simulink model "Luanvancu"  (R2018a)
settings: Solver=ode4  StartTime=0.0  StopTime=500  FixedStep=0.1  RelTol=1e-3
libraries: simulink x2
settings Model: EnablePacing=on  Creator=Hungs  LastModifiedBy=Hungs
settings DataIOCC: SaveOutput=off  SignalLogging=off  DSMLogging=off  SaveTime=off

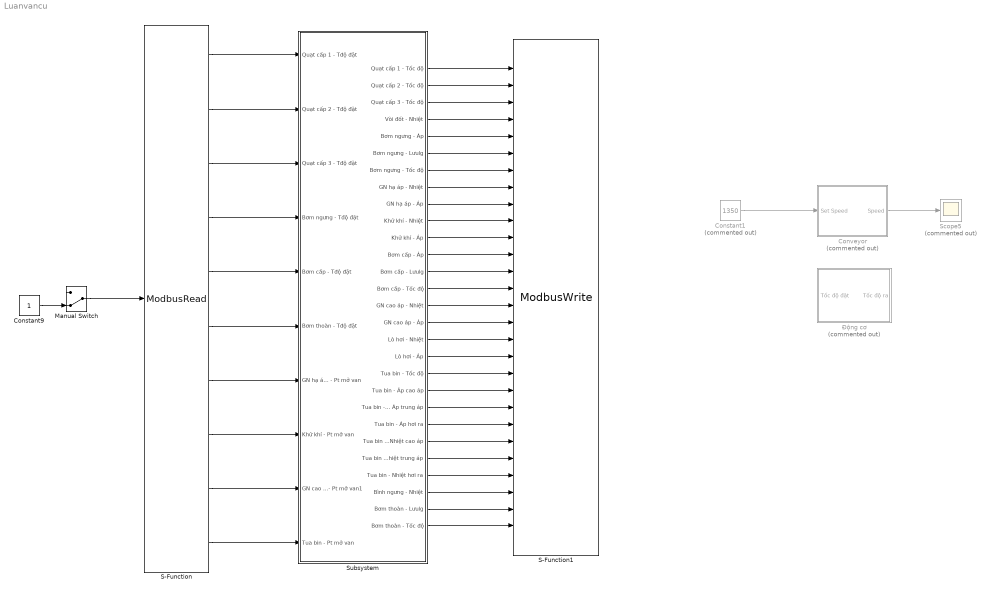
== system Luanvancu ==
  Constant1 : Constant  Commented=on  Value=1350
  Constant9 : Constant
  Conveyor : Subsystem  Commented=on
      mask Display: image('C:\Program Files\MATLAB\ThermalElectricity\Maskicon\conveyor.png');
  Manual Switch : ManualSwitch  CurrentSetting=0
  S-Function : S-Function  FunctionName=ModbusRead  Parameters='127.0.0.1' 502  SFunctionDeploymentMode=off  EnableBusSupport=off
  S-Function1 : S-Function  FunctionName=ModbusWrite  Parameters='127.0.0.1' 502  SFunctionDeploymentMode=off  EnableBusSupport=off
  Scope5 : Scope  Commented=on
  Subsystem : Subsystem
  Động cơ : Subsystem  Commented=on
  wires:
  Constant1/1 -> Conveyor/1(Set Speed)
  Conveyor/1(Speed) -> Scope5/1
  Manual Switch/1 -> S-Function/1
  Constant9/1 -> Manual Switch/2
  S-Function/1 -> Subsystem/1(Quạt cấp 1 - Tđộ đặt)
  S-Function/2 -> Subsystem/2(Quạt cấp 2 - Tđộ đặt)
  S-Function/3 -> Subsystem/3(Quạt cấp 3 - Tđộ đặt)
  S-Function/4 -> Subsystem/4(Bơm ngưng - Tđộ đặt)
  S-Function/5 -> Subsystem/5(Bơm cấp - Tđộ đặt)
  S-Function/6 -> Subsystem/6(Bơm thoàn - Tđộ đặt)
  S-Function/7 -> Subsystem/7(GN hạ áp - Pt mở van)
  S-Function/8 -> Subsystem/8(Khử khí - Pt mở van)
  S-Function/9 -> Subsystem/9(GN cao áp - Pt mở van1)
  S-Function/10 -> Subsystem/10(Tua bin - Pt mở van)
  Subsystem/1(Quạt cấp 1 - Tốc độ) -> S-Function1/1
  Subsystem/2(Quạt cấp 2 - Tốc độ) -> S-Function1/2
  Subsystem/3(Quạt cấp 3 - Tốc độ) -> S-Function1/3
  Subsystem/4(Vòi đốt - Nhiệt) -> S-Function1/4
  Subsystem/5(Bơm ngưng - Áp) -> S-Function1/5
  Subsystem/6(Bơm ngưng - Lưulg) -> S-Function1/6
  Subsystem/7(Bơm ngưng - Tốc độ) -> S-Function1/7
  Subsystem/8(GN hạ áp - Nhiệt) -> S-Function1/8
  Subsystem/9(GN hạ áp - Áp) -> S-Function1/9
  Subsystem/10(Khử khí - Nhiệt) -> S-Function1/10
  Subsystem/11(Khử khí - Áp) -> S-Function1/11
  Subsystem/12(Bơm cấp - Áp) -> S-Function1/12
  Subsystem/13(Bơm cấp - Lưulg) -> S-Function1/13
  Subsystem/14(Bơm cấp - Tốc độ) -> S-Function1/14
  Subsystem/15(GN cao áp - Nhiệt) -> S-Function1/15
  Subsystem/16(GN cao áp - Áp) -> S-Function1/16
  Subsystem/17(Lò hơi - Nhiệt) -> S-Function1/17
  Subsystem/18(Lò hơi - Áp) -> S-Function1/18
  Subsystem/19(Tua bin - Tốc độ) -> S-Function1/19
  Subsystem/20(Tua bin - Áp cao áp) -> S-Function1/20
  Subsystem/21(Tua bin - Áp trung áp) -> S-Function1/21
  Subsystem/22(Tua bin - Áp hơi ra) -> S-Function1/22
  Subsystem/23(Tua bin - Nhiệt cao áp) -> S-Function1/23
  Subsystem/24(Tua bin - Nhiệt trung áp) -> S-Function1/24
  Subsystem/25(Tua bin - Nhiệt hơi ra) -> S-Function1/25
  Subsystem/26(Bình ngưng - Nhiệt) -> S-Function1/26
  Subsystem/27(Bơm thoàn - Lưulg) -> S-Function1/27
  Subsystem/28(Bơm thoàn - Tốc độ) -> S-Function1/28

== system Luanvancu/Conveyor ==
  Set Speed : Inport
  Motor_1 : TransferFcn  Denominator=[1 1 1]
  Speed : Outport
  wires:
  Set Speed/1 -> Motor_1/1
  Motor_1/1 -> Speed/1

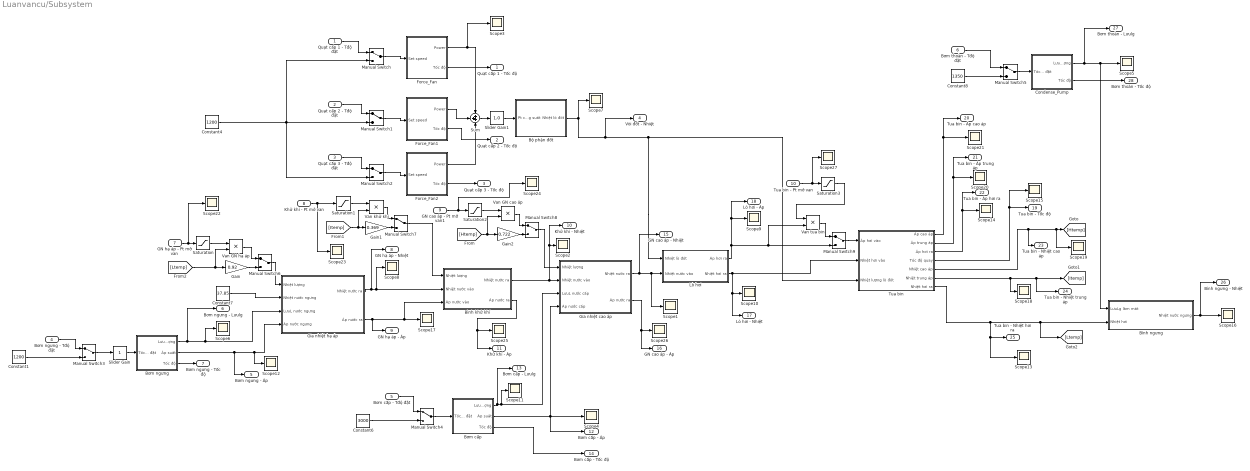
== system Luanvancu/Subsystem ==
  Quạt cấp 1 - Tđộ đặt : Inport
  Quạt cấp 2 - Tđộ đặt : Inport  Port=2
  Quạt cấp 3 - Tđộ đặt : Inport  Port=3
  Bơm ngưng - Tđộ đặt : Inport  Port=4
  Bơm cấp - Tđộ đặt : Inport  Port=5
  Bơm thoàn - Tđộ đặt : Inport  Port=6
  GN hạ áp - Pt mở van : Inport  Port=7
  Khử khí - Pt mở van : Inport  Port=8
  GN cao áp - Pt mở van1 : Inport  Port=9
  Tua bin - Pt mở van : Inport  Port=10
  Bình khử khí : Subsystem
  Bình ngưng : Subsystem
  Bơm cấp : Subsystem
      mask Display: image('C:\Program Files\MATLAB\ThermalElectricity\Maskicon\Pump.png');
  Bơm ngưng : Subsystem
      mask Display: image('C:\Program Files\MATLAB\ThermalElectricity\Maskicon\Pump.png');
  Bộ phận đốt : Subsystem
      mask Display: image('C:\Program Files\MATLAB\ThermalElectricity\Maskicon\Furnace.png');
  Condense_Pump : Subsystem
      mask Display: image('C:\Program Files\MATLAB\ThermalElectricity\Maskicon\Pump.png');
  Constant1 : Constant  Value=1200
  Constant4 : Constant  Value=1200
  Constant6 : Constant  Value=3000
  Constant7 : Constant  Value=37.85
  Constant8 : Constant  Value=1350
  Force_Fan : Subsystem
      mask Display: image('C:\Program Files\MATLAB\ThermalElectricity\Maskicon\Fan.png');
  Force_Fan1 : Subsystem
      mask Display: image('C:\Program Files\MATLAB\ThermalElectricity\Maskicon\Fan.png');
  Force_Fan2 : Subsystem
      mask Display: image('C:\Program Files\MATLAB\ThermalElectricity\Maskicon\Fan.png');
  Gain : Gain  Gain=0.92
  Gain1 : Gain  Gain=0.369
  Gain2 : Gain  Gain=0.722
  Gia nhiệt cao áp : Subsystem
  Gia nhiệt hạ áp : Subsystem
  Lò hơi : Subsystem
  Manual Switch{,1..9} (10 alike) : ManualSwitch
  Saturation{,1..3} (4 alike) : Saturate  UpperLimit=1  LowerLimit=0
  Scope{1..27} (27 alike) : Scope
  Slider Gain : simulink/Math Operations/Slider Gain  gain=1  low=0  high=2
  Slider Gain1 : simulink/Math Operations/Slider Gain  gain=1.0  low=0  high=2
  Sum : Sum  Inputs=+++
  Tua bin : Subsystem
  Van GN cao áp : Product
  Van GN hạ áp : Product
  Van khử khí : Product
  Van tua bin : Product
  Quạt cấp 1 - Tốc độ : Outport
  Quạt cấp 2 - Tốc độ : Outport  Port=2
  Quạt cấp 3 - Tốc độ : Outport  Port=3
  Vòi đốt - Nhiệt : Outport  Port=4
  Bơm ngưng - Áp : Outport  Port=5
  Bơm ngưng - Lưulg : Outport  Port=6
  Bơm ngưng - Tốc độ : Outport  Port=7
  GN hạ áp - Nhiệt : Outport  Port=8
  GN hạ áp - Áp : Outport  Port=9
  Khử khí - Nhiệt : Outport  Port=10
  Khử khí - Áp : Outport  Port=11
  Bơm cấp - Áp : Outport  Port=12
  Bơm cấp - Lưulg : Outport  Port=13
  Bơm cấp - Tốc độ : Outport  Port=14
  GN cao áp - Nhiệt : Outport  Port=15
  GN cao áp - Áp : Outport  Port=16
  Lò hơi - Nhiệt : Outport  Port=17
  Lò hơi - Áp : Outport  Port=18
  Tua bin - Tốc độ : Outport  Port=19
  Tua bin - Áp cao áp : Outport  Port=20
  Tua bin - Áp trung áp : Outport  Port=21
  Tua bin - Áp hơi ra : Outport  Port=22
  Tua bin - Nhiệt cao áp : Outport  Port=23
  Tua bin - Nhiệt trung áp : Outport  Port=24
  Tua bin - Nhiệt hơi ra : Outport  Port=25
  Bình ngưng - Nhiệt : Outport  Port=26
  Bơm thoàn - Lưulg : Outport  Port=27
  Bơm thoàn - Tốc độ : Outport  Port=28
  wires:
  Gia nhiệt cao áp/2(Áp nước ra) -> GN cao áp - Áp/1, Scope26/1
  Slider Gain1/1 -> Bộ phận đốt/1(Pt công suất)
  Sum/1 -> Slider Gain1/1
  Constant7/1 -> Gia nhiệt hạ áp/2(Nhiệt nước ngưng)
  Force_Fan/1(Power) -> Sum/1, Scope3/1
  Force_Fan1/1(Power) -> Sum/2
  Gia nhiệt hạ áp/2(Áp nước ra) -> GN hạ áp - Áp/1, Scope17/1, Bình khử khí/3(Áp nước vào)
  Lò hơi/1(Áp hơi ra) -> Lò hơi - Áp/1, Scope9/1, Manual Switch9/2, Van tua bin/2
  Bộ phận đốt/1(Nhiệt lò đốt) -> Vòi đốt - Nhiệt/1, Lò hơi/1(Nhiệt lò đốt), Tua bin/3(Nhiệt lượng lò đốt), Scope7/1
  Tua bin/3(Áp hơi ra) -> Tua bin - Áp hơi ra/1, Scope14/1
  Bình ngưng/1(Nhiệt nước ngưng) -> Bình ngưng - Nhiệt/1, Scope16/1
  Slider Gain/1 -> Bơm ngưng/1(Tốc độ đặt)
  Condense_Pump/1(Lưu lượng) -> Bơm thoàn - Lưulg/1, Bình ngưng/1(LưuLg làm mát), Scope5/1
  Bình khử khí/2(Áp nước ra) -> Khử khí - Áp/1, Scope25/1
  Tua bin/4(Tốc độ quay) -> Scope15/1, Tua bin - Tốc độ/1
  Manual Switch/1 -> Force_Fan/1(Set speed)
  Quạt cấp 1 - Tđộ đặt/1 -> Manual Switch/1
  Quạt cấp 2 - Tđộ đặt/1 -> Manual Switch1/1
  Manual Switch2/1 -> Force_Fan2/1(Set speed)
  Manual Switch1/1 -> Force_Fan1/1(Set speed)
  Quạt cấp 3 - Tđộ đặt/1 -> Manual Switch2/1
  Manual Switch3/1 -> Slider Gain/1
  Bơm ngưng - Tđộ đặt/1 -> Manual Switch3/1
  Manual Switch4/1 -> Bơm cấp/1(Tốc độ đặt)
  Bơm cấp - Tđộ đặt/1 -> Manual Switch4/1
  Manual Switch5/1 -> Condense_Pump/1(Tốc độ đặt)
  Constant8/1 -> Manual Switch5/2
  Bơm thoàn - Tđộ đặt/1 -> Manual Switch5/1
  Tua bin/6(Nhiệt trung áp) -> Scope18/1, Tua bin - Nhiệt trung áp/1, [Itemp]
  Tua bin/5(Nhiệt cao áp) -> Tua bin - Nhiệt cao áp/1, Scope19/1, [Htemp]
  [Ltemp] -> Van GN hạ áp/2, Gain/1
  Saturation/1 -> Van GN hạ áp/1
  Saturation1/1 -> Van khử khí/1
  [Htemp] -> Van GN cao áp/2, Gain2/1
  Saturation3/1 -> Van tua bin/1
  [Itemp] -> Van khử khí/2, Gain1/1
  Tua bin/7(Nhiệt hơi ra) -> Bình ngưng/2(Nhiệt hơi), [Ltemp], Scope13/1, Tua bin - Nhiệt hơi ra/1
  Bơm ngưng/1(Lưu lượng) -> Gia nhiệt hạ áp/3(LưuL nước ngưng), Scope6/1, Bơm ngưng - Lưulg/1
  Manual Switch6/1 -> Gia nhiệt hạ áp/1(Nhiệt lượng)
  Van GN hạ áp/1 -> Manual Switch6/1
  Manual Switch7/1 -> Bình khử khí/1(Nhiệt lượng)
  Van khử khí/1 -> Manual Switch7/1
  Manual Switch8/1 -> Gia nhiệt cao áp/1(Nhiệt lượng)
  Van GN cao áp/1 -> Manual Switch8/1
  Manual Switch9/1 -> Tua bin/1(Áp hơi vào)
  Van tua bin/1 -> Manual Switch9/1
  Bơm cấp/1(Lưu lượng) -> Bơm cấp - Lưulg/1, Scope11/1, Gia nhiệt cao áp/3(LưuL nước cấp)
  Gain/1 -> Manual Switch6/2
  Gain1/1 -> Manual Switch7/2
  Gain2/1 -> Manual Switch8/2
  Lò hơi/2(Nhiệt hơi ra) -> Lò hơi - Nhiệt/1, Scope10/1, Tua bin/2(Nhiệt hơi vào)
  Bơm ngưng/3(Tốc độ) -> Bơm ngưng - Tốc độ/1
  Bơm cấp/3(Tốc độ) -> Bơm cấp - Tốc độ/1
  Condense_Pump/2(Tốc độ) -> Bơm thoàn - Tốc độ/1
  Tua bin/2(Áp trung áp) -> Tua bin - Áp trung áp/1, Scope20/1
  Tua bin/1(Áp cao áp) -> Tua bin - Áp cao áp/1, Scope21/1
  Force_Fan2/1(Power) -> Sum/3
  Force_Fan2/2(Tốc độ) -> Quạt cấp 3 - Tốc độ/1
  Force_Fan1/2(Tốc độ) -> Quạt cấp 2 - Tốc độ/1
  Force_Fan/2(Tốc độ) -> Quạt cấp 1 - Tốc độ/1
  GN hạ áp - Pt mở van/1 -> Scope22/1, Saturation/1
  Bơm ngưng/2(Áp suất) -> Bơm ngưng - Áp/1, Scope12/1, Gia nhiệt hạ áp/4(Áp nước ngưng)
  Constant1/1 -> Manual Switch3/2
  Bơm cấp/2(Áp suất) -> Bơm cấp - Áp/1, Gia nhiệt cao áp/4(Áp nước cấp), Scope4/1
  Constant6/1 -> Manual Switch4/2
  Bình khử khí/1(Nhiệt nước ra) -> Khử khí - Nhiệt/1, Scope2/1, Gia nhiệt cao áp/2(Nhiệt nước vào)
  Gia nhiệt hạ áp/1(Nhiệt nước ra) -> GN hạ áp - Nhiệt/1, Bình khử khí/2(Nhiệt nước vào), Scope8/1
  Constant4/1 -> Manual Switch2/2, Manual Switch1/2, Manual Switch/2
  Gia nhiệt cao áp/1(Nhiệt nước ra) -> GN cao áp - Nhiệt/1, Scope1/1, Lò hơi/2(Nhiệt nước vào)
  Saturation2/1 -> Van GN cao áp/1
  GN cao áp - Pt mở van1/1 -> Scope24/1, Saturation2/1
  Khử khí - Pt mở van/1 -> Scope23/1, Saturation1/1
  Tua bin - Pt mở van/1 -> Scope27/1, Saturation3/1

== system Luanvancu/Động cơ ==
  Tốc độ đặt : Inport
  Bão hòa 2 cực : Saturate  UpperLimit=1500  LowerLimit=0
  Động cơ AC : TransferFcn  Denominator=[1 1 1]
  Tốc độ ra : Outport
  wires:
  Bão hòa 2 cực/1 -> Tốc độ ra/1
  Tốc độ đặt/1 -> Động cơ AC/1
  Động cơ AC/1 -> Bão hòa 2 cực/1

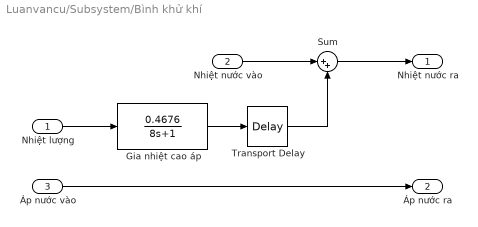
== system Luanvancu/Subsystem/Bình khử khí ==
  Nhiệt lượng : Inport
  Nhiệt nước vào : Inport  Port=2
  Áp nước vào : Inport  Port=3
  Gia nhiệt cao áp : TransferFcn  Numerator=[0.4676]  Denominator=[8 1]
  Sum : Sum  Inputs=|++
  Transport Delay : TransportDelay  DelayTime=3
  Nhiệt nước ra : Outport
  Áp nước ra : Outport  Port=2
  wires:
  Nhiệt lượng/1 -> Gia nhiệt cao áp/1
  Nhiệt nước vào/1 -> Sum/1
  Gia nhiệt cao áp/1 -> Transport Delay/1
  Sum/1 -> Nhiệt nước ra/1
  Áp nước vào/1 -> Áp nước ra/1
  Transport Delay/1 -> Sum/2

== system Luanvancu/Subsystem/Bình ngưng ==
  LưuLg làm mát : Inport
  Nhiệt hơi : Inport  Port=2
  Constant8 : Constant  Value=37.85
  Ngưng tụ : TransferFcn  Numerator=[6.883]  Denominator=[12 1]
  Sum : Sum  Inputs=|+-
  Sum1 : Sum  Inputs=|++
  Transport Delay : TransportDelay  DelayTime=3
  Nhiệt nước ngưng : Outport
  wires:
  Ngưng tụ/1 -> Transport Delay/1
  Nhiệt hơi/1 -> Sum/1
  LưuLg làm mát/1 -> Ngưng tụ/1
  Sum/1 -> Sum1/1
  Sum1/1 -> Nhiệt nước ngưng/1
  Constant8/1 -> Sum1/2
  Transport Delay/1 -> Sum/2

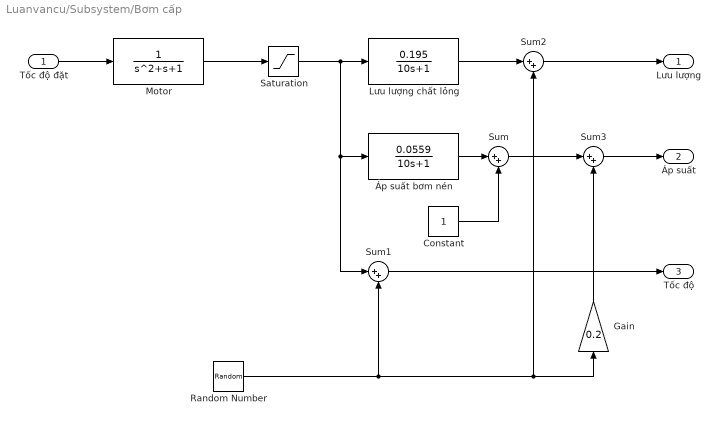
== system Luanvancu/Subsystem/Bơm cấp ==
  Tốc độ đặt : Inport
  Constant : Constant
  Gain : Gain  Gain=0.2
  Lưu lượng chất lỏng : TransferFcn  Numerator=[0.195]  Denominator=[10 1]
  Motor : TransferFcn  Denominator=[1 1 1]
  Random Number : RandomNumber  Variance=5  SampleTime=0.1
  Saturation : Saturate  UpperLimit=5645  LowerLimit=-5645
  Sum{,1..3} (4 alike) : Sum  Inputs=|++
  Áp suất bơm nén : TransferFcn  Numerator=[0.0559]  Denominator=[10 1]
  Lưu lượng : Outport
  Áp suất : Outport  Port=2
  Tốc độ : Outport  Port=3
  wires:
  Motor/1 -> Saturation/1
  Tốc độ đặt/1 -> Motor/1
  Áp suất bơm nén/1 -> Sum/1
  Constant/1 -> Sum/2
  Saturation/1 -> Lưu lượng chất lỏng/1, Sum1/1, Áp suất bơm nén/1
  Gain/1 -> Sum3/2
  Random Number/1 -> Gain/1, Sum2/2, Sum1/2
  Sum1/1 -> Tốc độ/1
  Lưu lượng chất lỏng/1 -> Sum2/1
  Sum2/1 -> Lưu lượng/1
  Sum/1 -> Sum3/1
  Sum3/1 -> Áp suất/1

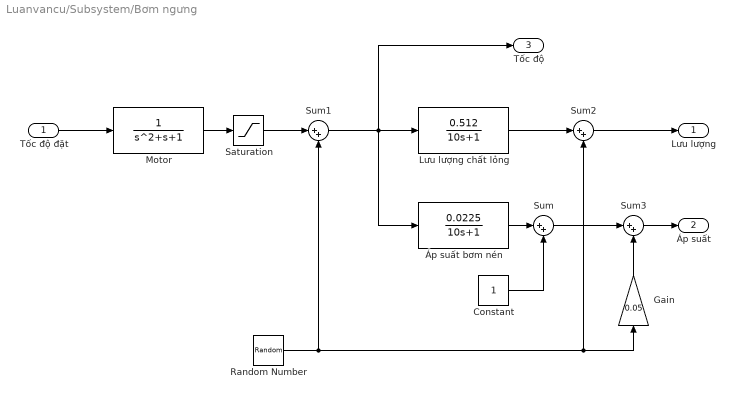
== system Luanvancu/Subsystem/Bơm ngưng ==
  Tốc độ đặt : Inport
  Constant : Constant
  Gain : Gain  Gain=0.05
  Lưu lượng chất lỏng : TransferFcn  Numerator=[0.512]  Denominator=[10 1]
  Motor : TransferFcn  Denominator=[1 1 1]
  Random Number : RandomNumber  Variance=5  SampleTime=0.1
  Saturation : Saturate  UpperLimit=1485  LowerLimit=-1485
  Sum{,1..3} (4 alike) : Sum  Inputs=|++
  Áp suất bơm nén : TransferFcn  Numerator=[0.0225]  Denominator=[10 1]
  Lưu lượng : Outport
  Áp suất : Outport  Port=2
  Tốc độ : Outport  Port=3
  wires:
  Tốc độ đặt/1 -> Motor/1
  Motor/1 -> Saturation/1
  Constant/1 -> Sum/2
  Áp suất bơm nén/1 -> Sum/1
  Sum1/1 -> Lưu lượng chất lỏng/1, Tốc độ/1, Áp suất bơm nén/1
  Random Number/1 -> Gain/1, Sum2/2, Sum1/2
  Saturation/1 -> Sum1/1
  Lưu lượng chất lỏng/1 -> Sum2/1
  Sum2/1 -> Lưu lượng/1
  Sum/1 -> Sum3/1
  Sum3/1 -> Áp suất/1
  Gain/1 -> Sum3/2

== system Luanvancu/Subsystem/Bộ phận đốt ==
  Pt công suất : Inport
  Transport Delay : TransportDelay  DelayTime=3
  Vòi đốt : TransferFcn  Numerator=[1687.5]  Denominator=[10 1]
  Nhiệt lò đốt : Outport
  wires:
  Vòi đốt/1 -> Transport Delay/1
  Pt công suất/1 -> Vòi đốt/1
  Transport Delay/1 -> Nhiệt lò đốt/1

== system Luanvancu/Subsystem/Condense_Pump ==
  Tốc độ đặt : Inport
  Condense_Flow : TransferFcn  Numerator=[0.012]  Denominator=[6 1]
  Motor : TransferFcn  Denominator=[1 1 1]
  Lưu lượng : Outport
  Tốc độ : Outport  Port=2
  wires:
  Motor/1 -> Tốc độ/1, Condense_Flow/1
  Tốc độ đặt/1 -> Motor/1
  Condense_Flow/1 -> Lưu lượng/1

== system Luanvancu/Subsystem/Force_Fan ==
  Set speed : Inport
  Heat_Power : TransferFcn  Numerator=[0.000222]  Denominator=[3 1]
  Motor : TransferFcn  Denominator=[1 1 1]
  Random Number : RandomNumber  Variance=5  SampleTime=0.1
  Saturation : Saturate  UpperLimit=1485  LowerLimit=-1485
  Sum1 : Sum  Inputs=|++
  Power : Outport
  Tốc độ : Outport  Port=2
  wires:
  Motor/1 -> Saturation/1
  Set speed/1 -> Motor/1
  Heat_Power/1 -> Power/1
  Random Number/1 -> Sum1/2
  Saturation/1 -> Sum1/1
  Sum1/1 -> Tốc độ/1, Heat_Power/1

== system Luanvancu/Subsystem/Force_Fan1 ==
  Set speed : Inport
  Heat_Power : TransferFcn  Numerator=[0.000222]  Denominator=[3 1]
  Motor : TransferFcn  Denominator=[1 1 1]
  Random Number : RandomNumber  Variance=5  SampleTime=0.1
  Saturation : Saturate  UpperLimit=1485  LowerLimit=-1485
  Sum1 : Sum  Inputs=|++
  Power : Outport
  Tốc độ : Outport  Port=2
  wires:
  Set speed/1 -> Motor/1
  Saturation/1 -> Sum1/1
  Sum1/1 -> Tốc độ/1, Heat_Power/1
  Motor/1 -> Saturation/1
  Heat_Power/1 -> Power/1
  Random Number/1 -> Sum1/2

== system Luanvancu/Subsystem/Force_Fan2 ==
  Set speed : Inport
  Heat_Power : TransferFcn  Numerator=[0.000222]  Denominator=[3 1]
  Motor : TransferFcn  Denominator=[1 1 1]
  Random Number : RandomNumber  Variance=5  SampleTime=0.1
  Saturation : Saturate  UpperLimit=1485  LowerLimit=-1485
  Sum1 : Sum  Inputs=|++
  Power : Outport
  Tốc độ : Outport  Port=2
  wires:
  Set speed/1 -> Motor/1
  Saturation/1 -> Sum1/1
  Sum1/1 -> Tốc độ/1, Heat_Power/1
  Motor/1 -> Saturation/1
  Heat_Power/1 -> Power/1
  Random Number/1 -> Sum1/2

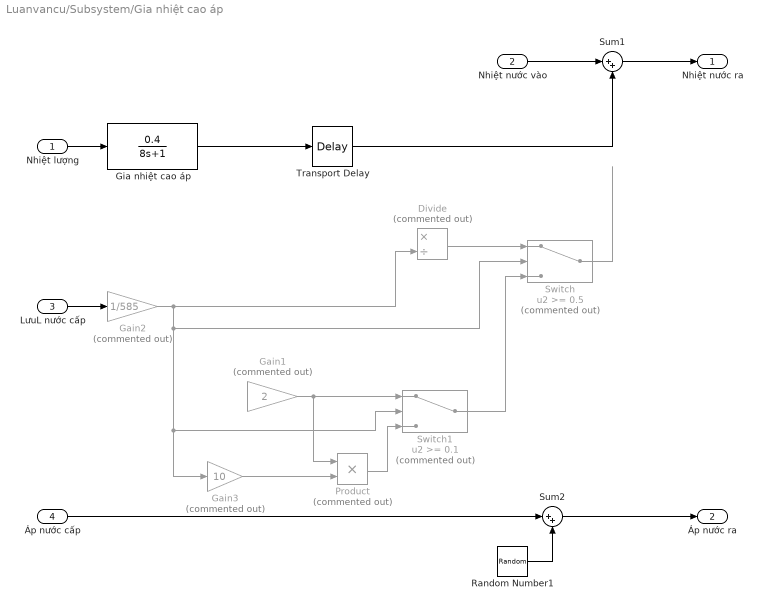
== system Luanvancu/Subsystem/Gia nhiệt cao áp ==
  Nhiệt lượng : Inport
  Nhiệt nước vào : Inport  Port=2
  LưuL nước cấp : Inport  Port=3
  Áp nước cấp : Inport  Port=4
  Divide : Product  Commented=on  Inputs=*/
  Gain1 : Gain  Commented=on  Gain=2
  Gain2 : Gain  Commented=on  Gain=1/585
  Gain3 : Gain  Commented=on  Gain=10
  Gia nhiệt cao áp : TransferFcn  Numerator=[0.4]  Denominator=[8 1]
  Product : Product  Commented=on
  Random Number1 : RandomNumber  SampleTime=0.1
  Sum1 : Sum  Inputs=|++
  Sum2 : Sum  Inputs=|++
  Switch : Switch  Commented=on  Threshold=0.5
  Switch1 : Switch  Commented=on  Threshold=0.1
  Transport Delay : TransportDelay  DelayTime=3
  Nhiệt nước ra : Outport
  Áp nước ra : Outport  Port=2
  wires:
  Nhiệt lượng/1 -> Gia nhiệt cao áp/1
  Switch1/1 -> Switch/3
  Sum1/1 -> Nhiệt nước ra/1
  Switch/1 -> ?
  Nhiệt nước vào/1 -> Sum1/1
  Gain1/1 -> Switch1/1, Product/1
  Gain3/1 -> Product/2
  Product/1 -> Switch1/3
  ? -> Divide/1, Gain1/1
  Gain2/1 -> Gain3/1, Switch1/2, Switch/2, Divide/2
  LưuL nước cấp/1 -> Gain2/1
  Divide/1 -> Switch/1
  Gia nhiệt cao áp/1 -> Transport Delay/1
  Transport Delay/1 -> Sum1/2
  Random Number1/1 -> Sum2/2
  Áp nước cấp/1 -> Sum2/1
  Sum2/1 -> Áp nước ra/1

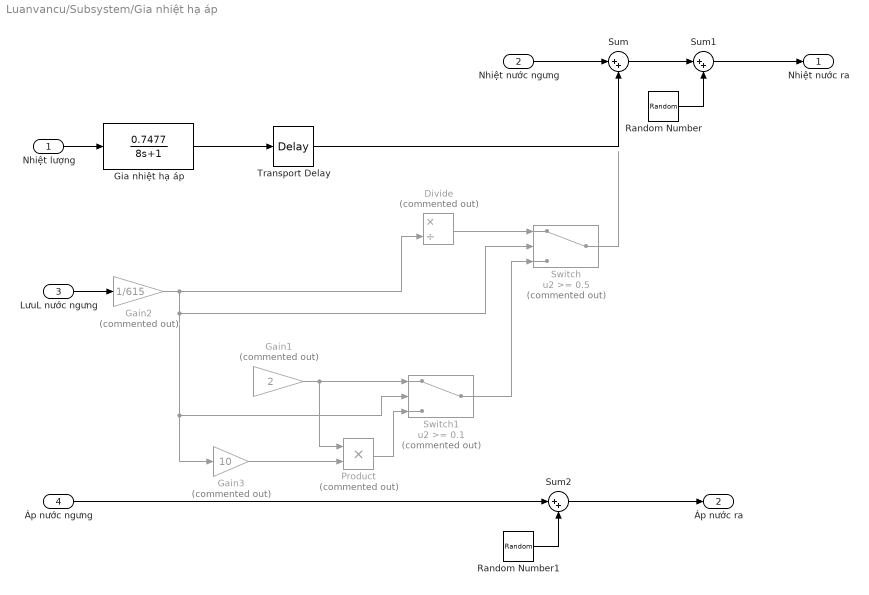
== system Luanvancu/Subsystem/Gia nhiệt hạ áp ==
  Nhiệt lượng : Inport
  Nhiệt nước ngưng : Inport  Port=2
  LưuL nước ngưng : Inport  Port=3
  Áp nước ngưng : Inport  Port=4
  Divide : Product  Commented=on  Inputs=*/
  Gain1 : Gain  Commented=on  Gain=2
  Gain2 : Gain  Commented=on  Gain=1/615
  Gain3 : Gain  Commented=on  Gain=10
  Gia nhiệt hạ áp : TransferFcn  Numerator=[0.7477]  Denominator=[8 1]
  Product : Product  Commented=on
  Random Number : RandomNumber  Variance=0.25  SampleTime=0.1
  Random Number1 : RandomNumber  Variance=0.25  SampleTime=0.1
  Sum : Sum  Inputs=|++
  Sum1 : Sum  Inputs=|++
  Sum2 : Sum  Inputs=|++
  Switch : Switch  Commented=on  Threshold=0.5
  Switch1 : Switch  Commented=on  Threshold=0.1
  Transport Delay : TransportDelay  DelayTime=3
  Nhiệt nước ra : Outport
  Áp nước ra : Outport  Port=2
  wires:
  Nhiệt nước ngưng/1 -> Sum/1
  Nhiệt lượng/1 -> Gia nhiệt hạ áp/1
  ? -> Divide/1, Gain1/1
  Gain2/1 -> Gain3/1, Switch1/2, Switch/2, Divide/2
  Gain1/1 -> Switch1/1, Product/1
  Switch1/1 -> Switch/3
  Gain3/1 -> Product/2
  Product/1 -> Switch1/3
  Divide/1 -> Switch/1
  Switch/1 -> ?
  LưuL nước ngưng/1 -> Gain2/1
  Gia nhiệt hạ áp/1 -> Transport Delay/1
  Transport Delay/1 -> Sum/2
  Sum/1 -> Sum1/1
  Sum1/1 -> Nhiệt nước ra/1
  Random Number/1 -> Sum1/2
  Áp nước ngưng/1 -> Sum2/1
  Sum2/1 -> Áp nước ra/1
  Random Number1/1 -> Sum2/2

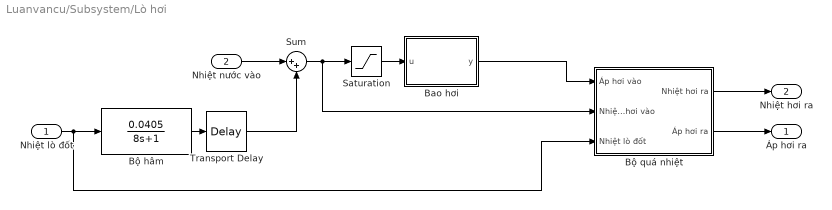
== system Luanvancu/Subsystem/Lò hơi ==
  Nhiệt lò đốt : Inport
  Nhiệt nước vào : Inport  Port=2
  Bao hơi : MATLAB Function  TreatAsAtomicUnit=on
  Bộ hâm : TransferFcn  Numerator=[0.0405]  Denominator=[8 1]
  Bộ quá nhiệt : Subsystem
  Saturation : Saturate  UpperLimit=425  LowerLimit=0
  Sum : Sum  Inputs=|++
  Transport Delay : TransportDelay  DelayTime=3
  Áp hơi ra : Outport
  Nhiệt hơi ra : Outport  Port=2
  wires:
  Sum/1 -> Bộ quá nhiệt/2(Nhiệt hơi vào), Saturation/1
  Nhiệt nước vào/1 -> Sum/1
  Nhiệt lò đốt/1 -> Bộ quá nhiệt/3(Nhiệt lò đốt), Bộ hâm/1
  Bộ quá nhiệt/1(Nhiệt hơi ra) -> Nhiệt hơi ra/1
  Saturation/1 -> Bao hơi/1(u)
  Bộ quá nhiệt/2(Áp hơi ra) -> Áp hơi ra/1
  Bộ hâm/1 -> Transport Delay/1
  Transport Delay/1 -> Sum/2
  Bao hơi/1(y) -> Bộ quá nhiệt/1(Áp hơi vào)

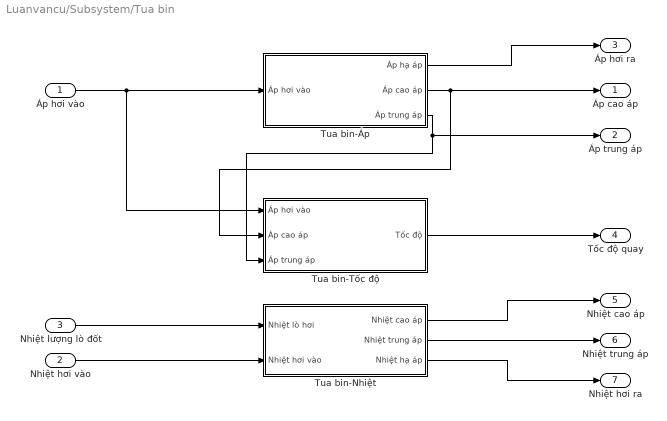
== system Luanvancu/Subsystem/Tua bin ==
  Áp hơi vào : Inport
  Nhiệt hơi vào : Inport  Port=2
  Nhiệt lượng lò đốt : Inport  Port=3
  Tua bin-Nhiệt : Subsystem
  Tua bin-Tốc độ : Subsystem
  Tua bin-Áp : Subsystem
  Áp cao áp : Outport
  Áp trung áp : Outport  Port=2
  Áp hơi ra : Outport  Port=3
  Tốc độ quay : Outport  Port=4
  Nhiệt cao áp : Outport  Port=5
  Nhiệt trung áp : Outport  Port=6
  Nhiệt hơi ra : Outport  Port=7
  wires:
  Tua bin-Áp/3(Áp trung áp) -> Tua bin-Tốc độ/3(Áp trung áp), Áp trung áp/1
  Tua bin-Áp/2(Áp cao áp) -> Tua bin-Tốc độ/2(Áp cao áp), Áp cao áp/1
  Áp hơi vào/1 -> Tua bin-Tốc độ/1(Áp hơi vào), Tua bin-Áp/1(Áp hơi vào)
  Nhiệt hơi vào/1 -> Tua bin-Nhiệt/2(Nhiệt hơi vào)
  Tua bin-Nhiệt/3(Nhiệt hạ áp) -> Nhiệt hơi ra/1
  Tua bin-Áp/1(Áp hạ áp) -> Áp hơi ra/1
  Tua bin-Tốc độ/1(Tốc độ) -> Tốc độ quay/1
  Nhiệt lượng lò đốt/1 -> Tua bin-Nhiệt/1(Nhiệt lò hơi)
  Tua bin-Nhiệt/1(Nhiệt cao áp) -> Nhiệt cao áp/1
  Tua bin-Nhiệt/2(Nhiệt trung áp) -> Nhiệt trung áp/1

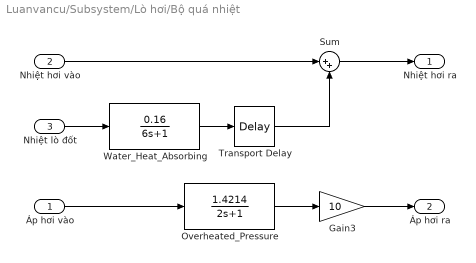
== system Luanvancu/Subsystem/Lò hơi/Bộ quá nhiệt ==
  Áp hơi vào : Inport
  Nhiệt hơi vào : Inport  Port=2
  Nhiệt lò đốt : Inport  Port=3
  Gain3 : Gain  Gain=10
  Overheated_Pressure : TransferFcn  Numerator=[1.4214]  Denominator=[2 1]
  Sum : Sum  Inputs=|++
  Transport Delay : TransportDelay
  Water_Heat_Absorbing : TransferFcn  Numerator=[0.16]  Denominator=[6 1]
  Nhiệt hơi ra : Outport
  Áp hơi ra : Outport  Port=2
  wires:
  Sum/1 -> Nhiệt hơi ra/1
  Water_Heat_Absorbing/1 -> Transport Delay/1
  Nhiệt hơi vào/1 -> Sum/1
  Nhiệt lò đốt/1 -> Water_Heat_Absorbing/1
  Áp hơi vào/1 -> Overheated_Pressure/1
  Overheated_Pressure/1 -> Gain3/1
  Gain3/1 -> Áp hơi ra/1
  Transport Delay/1 -> Sum/2

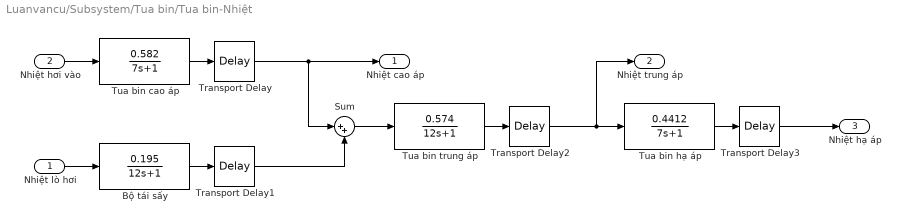
== system Luanvancu/Subsystem/Tua bin/Tua bin-Nhiệt ==
  Nhiệt lò hơi : Inport
  Nhiệt hơi vào : Inport  Port=2
  Bộ tái sấy : TransferFcn  Numerator=[0.195]  Denominator=[12 1]
  Sum : Sum  Inputs=|++
  Transport Delay : TransportDelay  DelayTime=2
  Transport Delay1 : TransportDelay  DelayTime=3
  Transport Delay2 : TransportDelay  DelayTime=2
  Transport Delay3 : TransportDelay  DelayTime=2
  Tua bin cao áp : TransferFcn  Numerator=[0.582]  Denominator=[7 1]
  Tua bin hạ áp : TransferFcn  Numerator=[0.4412]  Denominator=[7 1]
  Tua bin trung áp : TransferFcn  Numerator=[0.574]  Denominator=[12 1]
  Nhiệt cao áp : Outport
  Nhiệt trung áp : Outport  Port=2
  Nhiệt hạ áp : Outport  Port=3
  wires:
  Tua bin hạ áp/1 -> Transport Delay3/1
  Tua bin trung áp/1 -> Transport Delay2/1
  Sum/1 -> Tua bin trung áp/1
  Nhiệt hơi vào/1 -> Tua bin cao áp/1
  Bộ tái sấy/1 -> Transport Delay1/1
  Nhiệt lò hơi/1 -> Bộ tái sấy/1
  Tua bin cao áp/1 -> Transport Delay/1
  Transport Delay/1 -> Sum/1, Nhiệt cao áp/1
  Transport Delay1/1 -> Sum/2
  Transport Delay2/1 -> Nhiệt trung áp/1, Tua bin hạ áp/1
  Transport Delay3/1 -> Nhiệt hạ áp/1

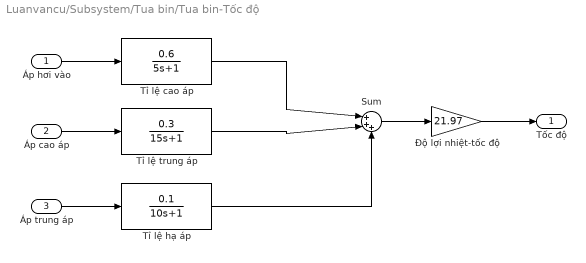
== system Luanvancu/Subsystem/Tua bin/Tua bin-Tốc độ ==
  Áp hơi vào : Inport
  Áp cao áp : Inport  Port=2
  Áp trung áp : Inport  Port=3
  Sum : Sum  Inputs=|+++
  Tỉ lệ cao áp : TransferFcn  Numerator=[0.6]  Denominator=[5 1]
  Tỉ lệ hạ áp : TransferFcn  Numerator=[0.1]  Denominator=[10 1]
  Tỉ lệ trung áp : TransferFcn  Numerator=[0.3]  Denominator=[15 1]
  Độ lợi nhiệt-tốc độ : Gain  Gain=21.97
  Tốc độ : Outport
  wires:
  Áp hơi vào/1 -> Tỉ lệ cao áp/1
  Tỉ lệ cao áp/1 -> Sum/1
  Sum/1 -> Độ lợi nhiệt-tốc độ/1
  Áp cao áp/1 -> Tỉ lệ trung áp/1
  Áp trung áp/1 -> Tỉ lệ hạ áp/1
  Tỉ lệ trung áp/1 -> Sum/2
  Tỉ lệ hạ áp/1 -> Sum/3
  Độ lợi nhiệt-tốc độ/1 -> Tốc độ/1

== system Luanvancu/Subsystem/Tua bin/Tua bin-Áp ==
  Áp hơi vào : Inport
  Tua bin cao áp : TransferFcn  Numerator=[0.18]  Denominator=[1 1]
  Tua bin hạ áp : TransferFcn  Numerator=[0.00757]  Denominator=[2 1]
  Tua bin trung áp : TransferFcn  Numerator=[0.2]  Denominator=[4 1]
  Áp hạ áp : Outport
  Áp cao áp : Outport  Port=2
  Áp trung áp : Outport  Port=3
  wires:
  Tua bin hạ áp/1 -> Áp hạ áp/1
  Tua bin trung áp/1 -> Áp trung áp/1, Tua bin hạ áp/1
  Tua bin cao áp/1 -> Áp cao áp/1, Tua bin trung áp/1
  Áp hơi vào/1 -> Tua bin cao áp/1

== matlab function Luanvancu/Subsystem/Lò hơi/Bao hơi ==
  data: u input; y output
function y = fcn(u)
to = [17 22 27 29.95 32.89 41.53 45.82 52.57 60.08 69.12 75.87 81.33 93.5 99.62 109.32 ...
    120.24 133.56 143.64 151.87 158.86 164.98 170.44 175.39 179.92 195.08 212.42 ...
    233.89 250.39 263.98 285.86 311.03 342.34 357.04 365.80 373.70 425];
p = [0.00192 0.00262 0.00354 0.004 0.005 0.008 0.01 0.018 0.02 0.03 0.04 0.05 0.08 0.1 0.14 0.2 0.3 0.4 ...
    0.5 0.6 0.7 0.8 0.9 1 1.4 2 3 4 5 7 10 15 18 20 22 35];
y = interp1(to,p,u);
